simulink model "EPS_tauhinput_simpletorquemap_simpletiremodel"  (R2022b)
settings: Solver=ode45  StartTime=0.0  StopTime=10.0  RelTol=1e-3  EnableMultiTasking=on
values from neighbouring files (symbols this model uses):
  amp_input_theta1 = amp_input_theta1_deg*pi/180    (= 1.0471975512)    [simulBack_theta1_simple.m]
  assist = 9.3    [simulBack_theta1_simple.m]
  C2 = 2.4    [simulBack_theta1_simple.m]
  Carspeed = 100    [simulBack_theta1_simple.m]
  deadband = 0    [simulBack_theta1_simple.m]
  freq_input_theta1 = 10    [simulBack_theta1_simple.m]
  friction_level = 0    [simulBack_theta1_simple.m]
  J1 = 0.033    [simulBack_theta1_simple.m]
  J2 = 0.085    [simulBack_theta1_simple.m]
  K = 143.24    [simulBack_theta1_simple.m]
  lagpole = 50    [simulBack_theta1_simple.m]
  lagzero = 15    [simulBack_theta1_simple.m]
  leadpole = 100    [simulBack_theta1_simple.m]
  leadzero = 10    [simulBack_theta1_simple.m]
  motor_onoff = 1    [simulBack_theta1_simple.m]
  motorcutoff = 100*2*3.14    (= 628)    [simulBack_theta1_simple.m]
  motordelay_onoff = 0    [simulBack_theta1_simple.m]
  offset_input_theta1 = 0    [simulBack_theta1_simple.m]
  tireangle_max = 60    [simulBack_theta1_simple.m]
settings Model: Creator=MSC-Dongwook  LastModifiedBy=LDW
settings SolverCC: AlgebraicLoopSolver=TrustRegion
settings DataIOCC: LimitDataPoints=on  SaveFormat=Array  ReturnWorkspaceOutputs=off
settings OptimizationCC: LifeSpan=inf
settings DebuggingCC: UnderspecifiedInitializationDetection=Classic  MergeDetectMultiDrivingBlocksExec=none  SolverPrmCheckMsg=warning  UnconnectedInputMsg=warning  UnconnectedOutputMsg=warning  UnconnectedLineMsg=warning  StateNameClashWarn=warning  SFUnexpectedBacktrackingDiag=warning  SFNoUnconditionalDefaultTransitionDiag=warning  SFExecutionAtInitializationDiag=none  SFMachineParentedDataDiag=warning  ArithmeticOperatorsInVariantConditions=warning
settings HardwareCC: ProdBitPerPointer=32  ProdBitPerSizeT=32  ProdBitPerPtrDiffT=32  ProdLargestAtomicFloat=None  ProdIntDivRoundTo=Undefined  ProdEndianess=Unspecified  ProdWordSize=32  ProdHWDeviceType=32-bit Generic
settings ModelReferenceCC: PropagateSignalLabelsOutOfModel=off
settings SFSimCC: SimUseLocalCustomCode=off  CustomCodeUndefinedFunction=UseInterfaceOnly
settings RTWCC: RTWUseLocalCustomCode=off
settings CodeAppCC: StateflowObjectComments=on
settings GRTTargetCC: TargetLangStandard=C89/C90 (ANSI)
settings ConfigComp: CovMetricSettings=dw  CovSaveCumulativeToWorkspaceVar=on  CovSaveSingleToWorkspaceVar=on  CovExternalEMLEnable=off

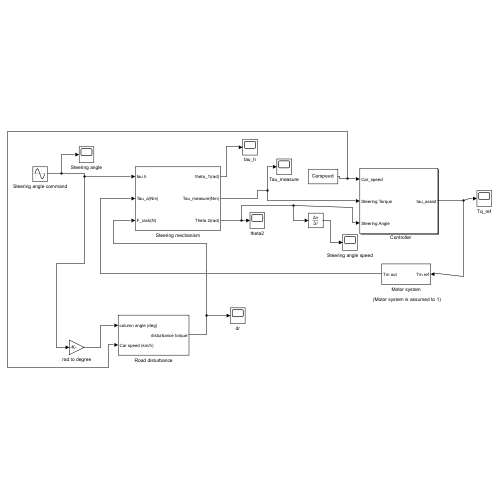
[thumbnail: Simulink's stored preview of the top-level diagram]
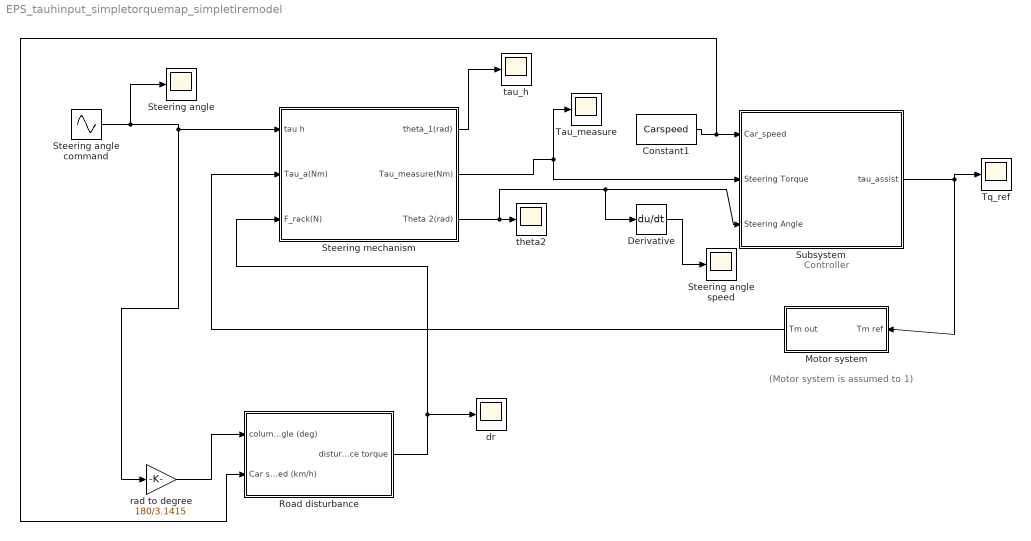
== system EPS_tauhinput_simpletorquemap_simpletiremodel ==
  note: Controller
  note: (Motor system is assumed to 1)
  Constant1 : Constant  Value=Carspeed
  Derivative : Derivative
  Motor system : Subsystem
  Road disturbance : Subsystem
  Steering angle : Scope
  Steering angle command : Sin  Amplitude=amp_input_theta1  Bias=offset_input_theta1  Frequency=freq_input_theta1*2*3.1415  SampleTime=0
  Steering angle speed : Scope
  Steering mechanism : Subsystem
  Subsystem : Subsystem
  Tau_measure : Scope
  Tq_ref : Scope
  dr : Scope
  rad to degree : Gain  Gain=180/3.1415
  tau_h : Scope
  theta2 : Scope
  wires:
  Steering mechanism/1(theta_1(rad)) -> tau_h/1
  Subsystem/1(tau_assist) -> Motor system/1(Tm ref), Tq_ref/1
  Steering mechanism/2(Tau_measure(Nm)) -> Subsystem/2(Steering Torque), Tau_measure/1
  Derivative/1 -> Steering angle speed/1
  Steering mechanism/3(Theta 2(rad)) -> Derivative/1, Subsystem/3(Steering Angle), theta2/1
  Steering angle command/1 -> Steering angle/1, Steering mechanism/1(tau h), rad to degree/1
  Constant1/1 -> Road disturbance/2(Car speed (km/h)), Subsystem/1(Car_speed)
  Motor system/1(Tm out) -> Steering mechanism/2(Tau_a(Nm))
  rad to degree/1 -> Road disturbance/1(column angle (deg))
  Road disturbance/1(disturbance torque) -> Steering mechanism/3(F_rack(N)), dr/1

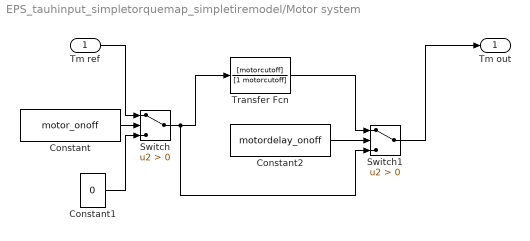
== system EPS_tauhinput_simpletorquemap_simpletiremodel/Motor system ==
  Tm ref : Inport
  Constant : Constant  Value=motor_onoff
  Constant1 : Constant  Value=0
  Constant2 : Constant  Value=motordelay_onoff
  Switch : Switch  Criteria=u2 > Threshold  SaturateOnIntegerOverflow=off  InputSameDT=off
  Switch1 : Switch  Criteria=u2 > Threshold  SaturateOnIntegerOverflow=off  InputSameDT=off
  Transfer Fcn : TransferFcn  Numerator=[motorcutoff]  Denominator=[1 motorcutoff]
  Tm out : Outport
  wires:
  Constant/1 -> Switch/2
  Tm ref/1 -> Switch/1
  Constant1/1 -> Switch/3
  Constant2/1 -> Switch1/2
  Switch1/1 -> Tm out/1
  Switch/1 -> Transfer Fcn/1, Switch1/3
  Transfer Fcn/1 -> Switch1/1

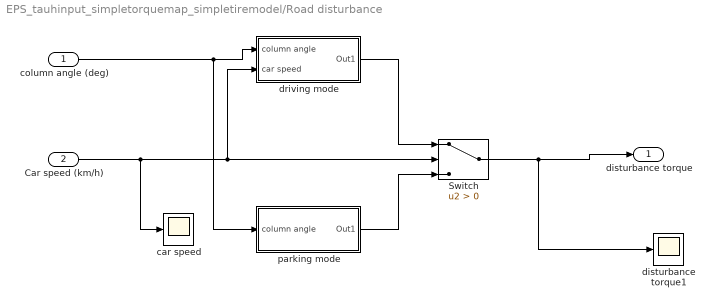
== system EPS_tauhinput_simpletorquemap_simpletiremodel/Road disturbance ==
  column angle (deg) : Inport
  Car speed (km/h) : Inport  Port=2
  Switch : Switch  Criteria=u2 > Threshold  SaturateOnIntegerOverflow=off  InputSameDT=off
  car speed : Scope
  disturbance torque1 : Scope
  driving mode : Subsystem
  parking mode : Subsystem
  disturbance torque : Outport
  wires:
  column angle (deg)/1 -> parking mode/1(column angle), driving mode/1(column angle)
  Car speed (km/h)/1 -> car speed/1, driving mode/2(car speed), Switch/2
  driving mode/1(Out1) -> Switch/1
  parking mode/1(Out1) -> Switch/3
  Switch/1 -> disturbance torque1/1, disturbance torque/1

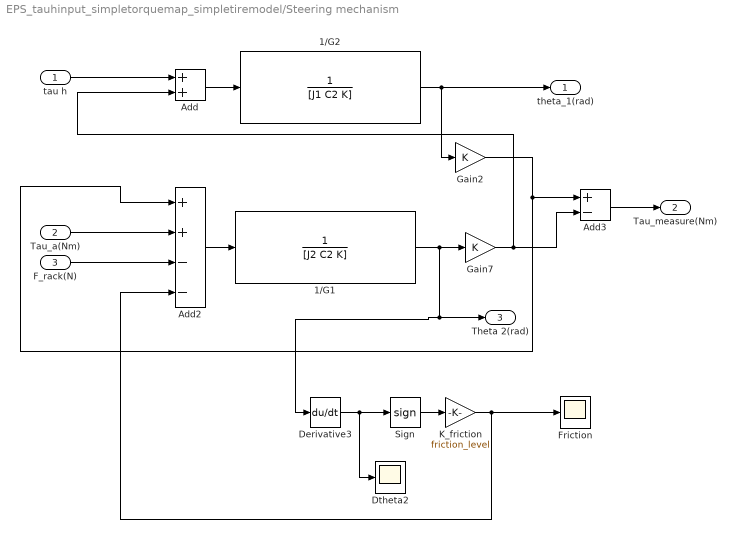
== system EPS_tauhinput_simpletorquemap_simpletiremodel/Steering mechanism ==
  tau h : Inport
  Tau_a(Nm) : Inport  Port=2
  F_rack(N) : Inport  Port=3
  1/G1 : TransferFcn  Denominator=[J2 C2 K]
  1/G2 : TransferFcn  Denominator=[J1 C2 K]
  Add : Sum
  Add2 : Sum  Inputs=++--
  Add3 : Sum  Inputs=+-
  Derivative3 : Derivative
  Dtheta2 : Scope
  Friction : Scope
  Gain2 : Gain  Gain=K
  Gain7 : Gain  Gain=K
  K_friction : Gain  Gain=friction_level
  Sign : Signum
  theta_1(rad) : Outport
  Tau_measure(Nm) : Outport  Port=2
  Theta 2(rad) : Outport  Port=3
  wires:
  tau h/1 -> Add/1
  Add/1 -> 1/G2/1
  1/G2/1 -> Gain2/1, theta_1(rad)/1
  Add2/1 -> 1/G1/1
  Tau_a(Nm)/1 -> Add2/2
  F_rack(N)/1 -> Add2/3
  1/G1/1 -> Derivative3/1, Theta 2(rad)/1, Gain7/1
  Gain2/1 -> Add3/1, Add2/1
  Gain7/1 -> Add/2, Add3/2
  Add3/1 -> Tau_measure(Nm)/1
  Derivative3/1 -> Dtheta2/1, Sign/1
  Sign/1 -> K_friction/1
  K_friction/1 -> Add2/4, Friction/1

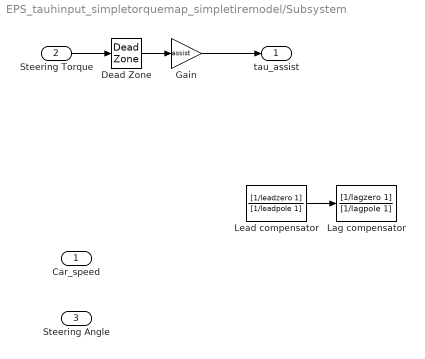
== system EPS_tauhinput_simpletorquemap_simpletiremodel/Subsystem ==
  Car_speed : Inport
  Steering Torque : Inport  Port=2
  Steering Angle : Inport  Port=3
  Dead Zone : DeadZone  LowerValue=-deadband  UpperValue=deadband
  Gain : Gain  Gain=assist
  Lag compensator : TransferFcn  Numerator=[1/lagzero 1]  Denominator=[1/lagpole 1]
  Lead compensator : TransferFcn  Numerator=[1/leadzero 1]  Denominator=[1/leadpole 1]
  tau_assist : Outport
  wires:
  Lead compensator/1 -> Lag compensator/1
  Steering Torque/1 -> Dead Zone/1
  Dead Zone/1 -> Gain/1
  Gain/1 -> tau_assist/1

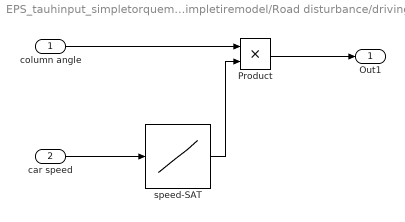
== system EPS_tauhinput_simpletorquemap_simpletiremodel/Road disturbance/driving mode ==
  column angle : Inport
  car speed : Inport  Port=2
  Product : Product
  speed-SAT : Lookup_n-D  NumberOfTableDimensions=1  BreakpointsForDimension1=[0,10,20,30,45,60,80]  Table=[0,0.057,0.082,0.132,0.25,0.385,0.673]  RndMeth=Simplest
  Out1 : Outport
  wires:
  speed-SAT/1 -> Product/2
  car speed/1 -> speed-SAT/1
  column angle/1 -> Product/1
  Product/1 -> Out1/1

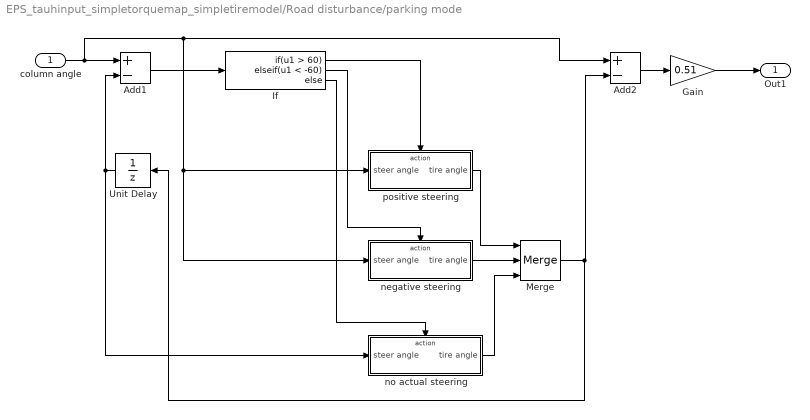
== system EPS_tauhinput_simpletorquemap_simpletiremodel/Road disturbance/parking mode ==
  column angle : Inport
  Add1 : Sum  Inputs=+-
  Add2 : Sum  Inputs=+-
  Gain : Gain  Gain=0.51
  If : If  IfExpression=u1 > 60  ElseIfExpressions=u1 < -60
  Merge : Merge  Inputs=3
  Unit Delay : UnitDelay  SampleTime=-1  HasFrameUpgradeWarning=on
  negative steering : Subsystem  TreatAsAtomicUnit=on
  no actual steering : Subsystem  TreatAsAtomicUnit=on
  positive steering : Subsystem  TreatAsAtomicUnit=on
  Out1 : Outport
  wires:
  column angle/1 -> positive steering/1(steer angle), negative steering/1(steer angle), Add2/1, Add1/1
  Add1/1 -> If/1
  If/1 -> positive steering/Action
  If/2 -> negative steering/Action
  If/3 -> no actual steering/Action
  Unit Delay/1 -> Add1/2, no actual steering/1(steer angle)
  positive steering/1(tire angle) -> Merge/1
  negative steering/1(tire angle) -> Merge/2
  no actual steering/1(tire angle) -> Merge/3
  Merge/1 -> Unit Delay/1, Add2/2
  Add2/1 -> Gain/1
  Gain/1 -> Out1/1

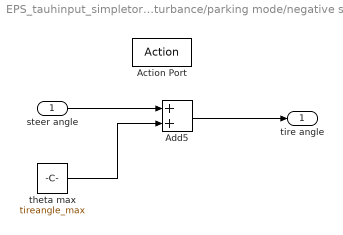
== system EPS_tauhinput_simpletorquemap_simpletiremodel/Road disturbance/parking mode/negative steering ==
  steer angle : Inport
  Action Port : ActionPort
  Add5 : Sum
  theta max : Constant  Value=tireangle_max
  tire angle : Outport
  wires:
  steer angle/1 -> Add5/1
  theta max/1 -> Add5/2
  Add5/1 -> tire angle/1

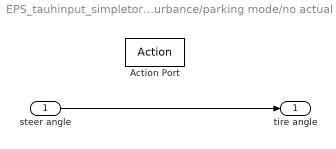
== system EPS_tauhinput_simpletorquemap_simpletiremodel/Road disturbance/parking mode/no actual steering ==
  steer angle : Inport
  Action Port : ActionPort
  tire angle : Outport
  wires:
  steer angle/1 -> tire angle/1

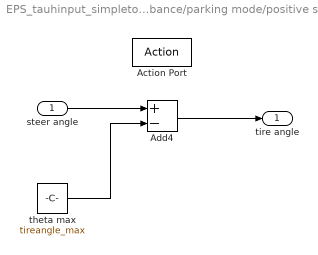
== system EPS_tauhinput_simpletorquemap_simpletiremodel/Road disturbance/parking mode/positive steering ==
  steer angle : Inport
  Action Port : ActionPort
  Add4 : Sum  Inputs=+-
  theta max : Constant  Value=tireangle_max
  tire angle : Outport
  wires:
  steer angle/1 -> Add4/1
  theta max/1 -> Add4/2
  Add4/1 -> tire angle/1
